simulink library "lib_EMachine"  (R2017b)
settings: Solver=VariableStepAuto  StartTime=0.0  StopTime=10.0  RelTol=1e-3
undefined symbols (not defined in the file): mot, t_amb, tloop
libraries: simulink x6, lib_Clutch x1
(part 2 of 2)

== system lib_EMachine/E-Machine/Soft MCU/Torque Calculation1/max torque /Heat index ==
  note: Heat index calculation
  cont torque : Inport
  torque : Inport  Port=2
  Abs : Abs  SaturateOnIntegerOverflow=on
  Divide : Subsystem  mask(Divide){}
      mask Display: disp('Divide')
  Heat Energy Factor : Integrator  InitialCondition=-0.3  LimitOutput=on  UpperSaturationLimit=1  LowerSaturationLimit=-0.3
  Heating Constant : Gain  Gain=0.3/mot.plant.init.t_max_trq  SaturateOnIntegerOverflow=on  OutDataTypeStr=Inherit: Same as input  ParamDataTypeStr=Inherit: Same as input
  Saturation : Saturate  UpperLimit=1  LowerLimit=0
  Sum : Sum  Inputs=+-  SaturateOnIntegerOverflow=on  InputSameDT=on  OutDataTypeStr=Inherit: Same as first input
  motor inertia (Nms^2\rad)5 : Constant
  Heat index : Outport
  wires:
  torque/1 -> Divide/1(numerator)
  Heat Energy Factor/1 -> Saturation/1
  Heating Constant/1 -> Heat Energy Factor/1
  Sum/1 -> Heating Constant/1
  Divide/1(quotient) -> Abs/1
  motor inertia (Nms^2\rad)5/1 -> Sum/2
  Saturation/1 -> Heat index/1
  Abs/1 -> Sum/1
  cont torque/1 -> Divide/2(denominator)

== system lib_EMachine/E-Machine/Soft MCU/Torque Calculation2/max torque /Divide by zero ==
  In1 : Inport
  Compare To Constant : simulink/Logic and Bit Operations/Compare To Constant  relop===  const=0  OutDataTypeStr=boolean
  Constant1 : Constant
  Switch2 : Switch  Criteria=u2 > Threshold
  Out1 : Outport
  wires:
  Switch2/1 -> Out1/1
  In1/1 -> Compare To Constant/1, Switch2/3
  Compare To Constant/1 -> Switch2/2
  Constant1/1 -> Switch2/1

== system lib_EMachine/E-Machine/Soft MCU/Torque Calculation2/max torque /Heat index ==
  note: Heat index calculation
  cont torque : Inport
  torque : Inport  Port=2
  Abs : Abs  SaturateOnIntegerOverflow=on
  Divide : Subsystem  mask(Divide){}
      mask Display: disp('Divide')
  Heat Energy Factor : Integrator  InitialCondition=-0.3  LimitOutput=on  UpperSaturationLimit=1  LowerSaturationLimit=-0.3
  Heating Constant : Gain  Gain=0.3/mot.plant.init.t_max_trq  SaturateOnIntegerOverflow=on  OutDataTypeStr=Inherit: Same as input  ParamDataTypeStr=Inherit: Same as input
  Saturation : Saturate  UpperLimit=1  LowerLimit=0
  Sum : Sum  Inputs=+-  SaturateOnIntegerOverflow=on  InputSameDT=on  OutDataTypeStr=Inherit: Same as first input
  motor inertia (Nms^2\rad)5 : Constant
  Heat index : Outport
  wires:
  torque/1 -> Divide/1(numerator)
  Heat Energy Factor/1 -> Saturation/1
  Heating Constant/1 -> Heat Energy Factor/1
  Sum/1 -> Heating Constant/1
  Divide/1(quotient) -> Abs/1
  motor inertia (Nms^2\rad)5/1 -> Sum/2
  Saturation/1 -> Heat index/1
  Abs/1 -> Sum/1
  cont torque/1 -> Divide/2(denominator)

== system lib_EMachine/E-Machine/IMG Plant/Electric Machine/Thermal1/MotInv_loop/MCUOverTemp Fault ==
  In1 : Inport
  Gain : Gain  Gain=3
  Switch : Switch  Threshold=1
  Out1 : Outport
  wires:
  In1/1 -> Switch/3, Gain/1
  [MCUOverTemp] -> Switch/2
  Gain/1 -> Switch/1
  Switch/1 -> Out1/1

== system lib_EMachine/E-Machine/IMG Plant/Electric Machine/Thermal1/MotInv_loop/MotorOverTempFault ==
  In1 : Inport
  Gain : Gain  Gain=2
  Memory : Memory
  Switch1 : Switch  Threshold=1
  Out1 : Outport
  wires:
  Memory/1 -> Gain/1
  In1/1 -> Memory/1, Switch1/3
  [MotOverTemp] -> Switch1/2
  Gain/1 -> Switch1/1
  Switch1/1 -> Out1/1

== system lib_EMachine/E-Machine/IMG Plant/Electric Machine/Thermal1/Motor Thermal/Lower Limit ==
  In1 : Inport
  Constant3 : Constant  Value=Lolimit
  MinMax : MinMax  Function=max  Inputs=2
  Out1 : Outport
  wires:
  In1/1 -> MinMax/1
  Constant3/1 -> MinMax/2
  MinMax/1 -> Out1/1

== system lib_EMachine/E-Machine/Soft MCU/Torque Calculation1/max torque /Heat index/Divide ==
  note: Take care of
      | division by 0
  numerator : Inport
  denominator : Inport  Port=2
  Fcn : Fcn  Expr=u[1] / ( u[2] + eps*(u[2]==0) )
  Mux : Mux  Inputs=2
  quotient : Outport
  wires:
  Mux/1 -> Fcn/1
  numerator/1 -> Mux/1
  Fcn/1 -> quotient/1
  denominator/1 -> Mux/2

== system lib_EMachine/E-Machine/Soft MCU/Torque Calculation2/max torque /Heat index/Divide ==
  note: Take care of
      | division by 0
  numerator : Inport
  denominator : Inport  Port=2
  Fcn : Fcn  Expr=u[1] / ( u[2] + eps*(u[2]==0) )
  Mux : Mux  Inputs=2
  quotient : Outport
  wires:
  Mux/1 -> Fcn/1
  numerator/1 -> Mux/1
  Fcn/1 -> quotient/1
  denominator/1 -> Mux/2

== matlab function lib_EMachine/E-Machine/Soft MCU/diff_INV_state ==
  data: u input; y output
function y = fcn(u)
if(u == 3) %when inverter is in standby state
    y = 0;
elseif(u == 8) %when inverter is in torque control state
    y = 1;
elseif(u==14) %when invertor is in error state
    y = 2;
else
    y = 0;
end

== matlab function lib_EMachine/E-Machine/Soft MCU/diff_INV_state1 ==
  data: u input; y output
function y = fcn(u)
if(u == 0) %when inverter is in standby state
    y = 0;
elseif(u == 1) %when inverter is in torque control state
    y = 1;
elseif(u==2) %when invertor is in error state
    y = 0;
else
    y = 0;
end
